simulink model "single_boat_simulation_R2018b"  (R2018b)
settings: Solver=VariableStepAuto  StartTime=0.0  StopTime=P.Tend  MaxStep=0.05  MinStep=0.001  RelTol=1e-3
InitFcn:
  | boat_init;
  | iD = 1;
StopFcn:
  | disp('finished sim')
  | boat_show_data;
  | disp('finished plot')
values from neighbouring files (symbols this model uses):
  Param = P    [boat_init.m]    (also in boat_init_mpc.m)
settings Model: SimulationMode=accelerator  Creator=Bruno  LastModifiedBy=Bruno
settings DataIOCC: ReturnWorkspaceOutputs=on
settings DebuggingCC: UnconnectedInputMsg=none  UnconnectedOutputMsg=none  UnconnectedLineMsg=none  SFMachineParentedDataDiag=error
settings ModelReferenceCC: EnableRefExpFcnMdlSchedulingChecks=off
settings RTWCC: Description=Generic Real-Time Target

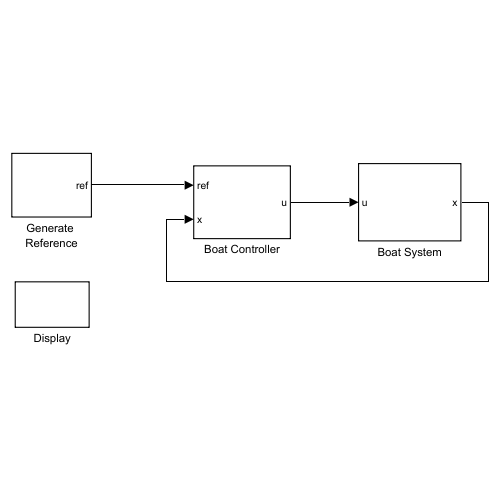
[thumbnail: Simulink's stored preview of the top-level diagram]
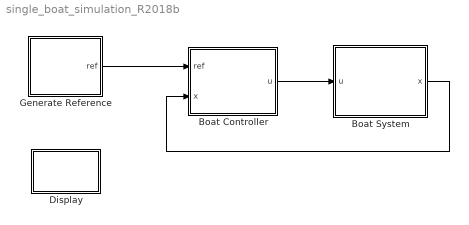
== system single_boat_simulation_R2018b ==
  Boat Controller : Subsystem
  Boat System : Subsystem
  Display : Subsystem
  Generate Reference : Subsystem
  wires:
  Generate Reference/1(ref) -> Boat Controller/1(ref)
  Boat System/1(x) -> Boat Controller/2(x)
  Boat Controller/1(u) -> Boat System/1(u)

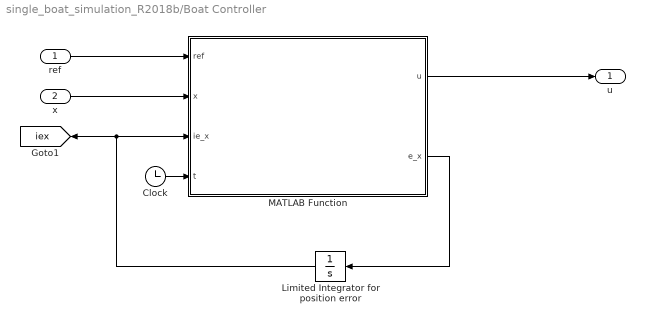
== system single_boat_simulation_R2018b/Boat Controller ==
  ref : Inport
  x : Inport  Port=2
  Clock : Clock
  Limited Integrator for position error : Integrator  LimitOutput=on  UpperSaturationLimit=100  LowerSaturationLimit=-100
  MATLAB Function : MATLAB Function  TreatAsAtomicUnit=on
  u : Outport
  tag scope: iex=global
  wires:
  MATLAB Function/2(e_x) -> Limited Integrator for position error/1
  MATLAB Function/1(u) -> u/1
  Limited Integrator for position error/1 -> MATLAB Function/3(ie_x), [iex]
  ref/1 -> MATLAB Function/1(ref)
  x/1 -> MATLAB Function/2(x)
  Clock/1 -> MATLAB Function/4(t)

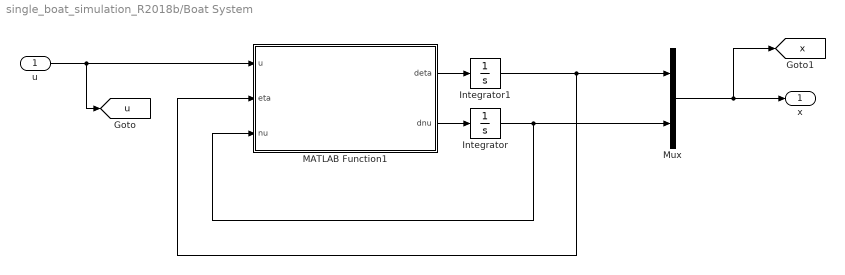
== system single_boat_simulation_R2018b/Boat System ==
  u : Inport
  Integrator : Integrator  InitialCondition=Param.nu0  ContinuousStateAttributes='v'
  Integrator1 : Integrator  InitialCondition=Param.eta0  ContinuousStateAttributes='p'
  MATLAB Function1 : MATLAB Function  TreatAsAtomicUnit=on
  Mux : Mux  Inputs=2
  x : Outport
  tag scope: u=global, x=global
  wires:
  Integrator/1 -> MATLAB Function1/3(nu), Mux/2
  MATLAB Function1/2(dnu) -> Integrator/1
  Integrator1/1 -> MATLAB Function1/2(eta), Mux/1
  MATLAB Function1/1(deta) -> Integrator1/1
  u/1 -> [u], MATLAB Function1/1(u)
  Mux/1 -> x/1, [x]

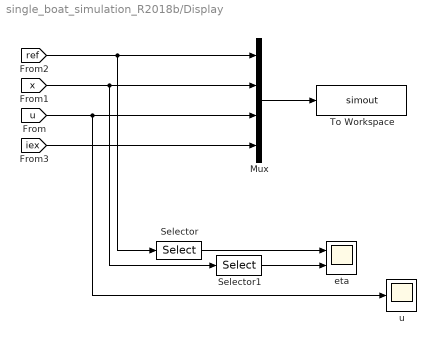
== system single_boat_simulation_R2018b/Display ==
  Mux : Mux
  Selector : Selector  InputPortWidth=6  IndexOptions=Index vector (dialog)  Indices=[1:3]  OutputSizes=1
  Selector1 : Selector  InputPortWidth=6  IndexOptions=Index vector (dialog)  Indices=[1:3]  OutputSizes=1
  To Workspace : ToWorkspace  VariableName=simout  SaveFormat=Structure With Time  SampleTime=-1
  eta : Scope  NumInputPorts=2
  u : Scope
  wires:
  [x] -> Selector1/1, Mux/2
  [u] -> u/1, Mux/3
  [iex] -> Mux/4
  [ref] -> Selector/1, Mux/1
  Mux/1 -> To Workspace/1
  Selector/1 -> eta/1
  Selector1/1 -> eta/2

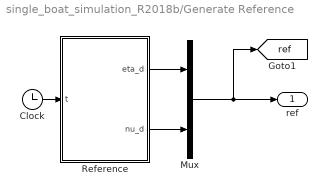
== system single_boat_simulation_R2018b/Generate Reference ==
  Clock : Clock
  Mux : Mux  Inputs=2
  Reference : MATLAB Function  TreatAsAtomicUnit=on
  ref : Outport
  tag scope: ref=global
  wires:
  Clock/1 -> Reference/1(t)
  Mux/1 -> [ref], ref/1
  Reference/1(eta_d) -> Mux/1
  Reference/2(nu_d) -> Mux/2

== matlab function single_boat_simulation_R2018b/Boat Controller/MATLAB Function ==
  data: ref input; x input; ie_x input; t input; u output; Param parameter; e_x output size=2
function [u,e_x] = controller(ref,x,ie_x,t,Param)
    
    eta = x(1:3,1);
    nu = x(4:6,1);
    eta_d = ref(1:3,1);
    nu_d = ref(4:6,1);

    [u,e_x] = boat_ctrl(eta,nu,Param,eta_d,nu_d,ie_x,t);

    
end

== matlab function single_boat_simulation_R2018b/Generate Reference/Reference ==
  data: t input; eta_d output; nu_d output; Param parameter
function [eta_d,nu_d] = get_ref(t,Param)
    
    [eta_d,nu_d] = get_boat_ref(t,Param);

end

== matlab function single_boat_simulation_R2018b/Boat System/MATLAB Function1 ==
  data: u input; deta output size=3; eta input; nu input; dnu output size=3; Param parameter
function [deta,dnu] = dynamics(u,eta,nu,Param)
    
    [deta,dnu] = boat_full_dyn(eta,nu,u,Param);
    
end
